simulink model "can_simple_block_bu11143"  (R2016b)
settings: Solver=FixedStepDiscrete  StartTime=0.0  StopTime=1000  FixedStep=0.2  RelTol=1e-3  EnableMultiTasking=on
undefined symbols (not defined in the file or in its folder): A, A10, A14, B, B11, B12, B13, B8, C, CS0, CS1, D, D11, D4, F3, F4, G, G3, G4, H3, H4, K17, K4, L3, N16, PA11, PA12, PD0, PE14, PE15, R10, R14, R17, SCK, SIN, SOUT, T14
libraries: rappid_564xl_ec_toolbox x59
(part 3 of 6)

== matlab function can_simple_block_bu11143/Function-Call Subsystem/Subsystem2/RawData to StoreData ==
  data: StrCell input; CellSOC_1_104 data_store_memory; VSOCDataCAN_8b output uint8
function VSOCDataCAN_8b = fcn(StrCell)

global CellSOC_1_104;
VSOCDataCAN_8b =  uint8(zeros(1,8));

      VSOCDataCAN_8b(1) =         CellSOC_1_104(StrCell*4-3)/256;
      VSOCDataCAN_8b(2) = mod(CellSOC_1_104(StrCell*4-3),256);
      VSOCDataCAN_8b(3) =         CellSOC_1_104(StrCell*4-2)/256;
      VSOCDataCAN_8b(4) = mod(CellSOC_1_104(StrCell*4-2),256);
      VSOCDataCAN_8b(5) =         CellSOC_1_104(StrCell*4-1)/256;
      VSOCDataCAN_8b(6) = mod(CellSOC_1_104(StrCell*4-1),256);
      VSOCDataCAN_8b(7) =         CellSOC_1_104(StrCell*4   )/256;
      VSOCDataCAN_8b(8) = mod(CellSOC_1_104(StrCell*4   ),256);

% VTDataCAN_8b(1) =         CellV_1_104(1)/256;
% VTDataCAN_8b(2) = mod(CellV_1_104(1),256);
% VTDataCAN_8b(3) =         CellV_1_104(2)/256;
% VTDataCAN_8b(4) = mod(CellV_1_104(2),256);
% VTDataCAN_8b(5) =         CellV_1_104(9)/256;
% VTDataCAN_8b(6) = mod(CellV_1_104(9),256);
% VTDataCAN_8b(7) =         CellV_1_104(10)/256;
% VTDataCAN_8b(8) = mod(CellV_1_104(10),256);

% VTDataCAN_8b(1) =         uint16(30000)/256;
% VTDataCAN_8b(2) = mod(uint16(30000),256);
% VTDataCAN_8b(3) =         uint16(35000)/256;
% VTDataCAN_8b(4) = mod(uint16(35000),256);
% VTDataCAN_8b(5) =         uint16(33000)/256;
% VTDataCAN_8b(6) = mod(uint16(33000),256);
% VTDataCAN_8b(7) =         uint16(20000)/256;
% VTDataCAN_8b(8) = mod(uint16(20000),256);


end








% CellV_1_104(1) = uint16(1);

% SPIDataStore = uint16(zeros(1,21));
% DataFault =  zeros(1,7);
%
% for i=1:7
%   SPIDataStore(i*3-2) = SPIData(i*8-7)+SPIData(i*8-6)*256;
%   SPIDataStore(i*3-1) = SPIData(i*8-5)+SPIData(i*8-4)*256;
%   SPIDataStore(i*3   ) = SPIData(i*8-3)+SPIData(i*8-2)*256;
%   if (PecChk(i*2-1) == SPIData(i*8-1)) && (PecChk(i*2) == SPIData(i*8))
%     DataFault(i) = 1;
%   else
%     DataFault(i) = 0;
%   end
% end



% onemask8 = uint16(hex2dec('00FF'));
% onemask8_8sft = uint16(hex2dec('FF00'));
% onemask88 = uint8(hex2dec('FF'));
% onemask16 = uint16(hex2dec('FFFF'));
%
% % data_test = zeros(1,2);
% remainder = uint16(16);
%
% for i=1:len
%     ii = uint16(i);
% %     data_test(1,i) = data(ii);
% %     address = 2;
%     address = bitand( ...
%         bitxor( ...
%         uint8(bitsra(remainder,7)),data(ii) ), ...
%         onemask88);
%     remainder = bitxor(bitshift(remainder,8,'uint16'),pec15Table(address+1));
% end
% pec15 = uint16(bitand(bitshift(remainder,1,'uint16'),onemask16));
% pec0 = uint8(bitand(pec15,onemask8));
% pec1 = uint8(bitsra(bitand(pec15,onemask8_8sft),8));

== stateflow chart can_simple_block_bu11143/Function-Call Subsystem/T_DUMP_CAN ==
  state A
    en: count = 0;
    du: count = count + 1;
  state A1
    en: count = 0;
  (default) -> A : {count =0;}
  A -> A1 : [count > count_in]{sig_trigger}
  A1 -> A
  data: count local double [0..10000]; count_in input
  events: sig_trigger output FUNCTION_CALL_EVENT

== stateflow chart can_simple_block_bu11143/Function-Call Subsystem/Subsystem4/Chart1 ==
  state A
    en: count  = count + 1;
    du: count = count + 1;
  state A1
    en: count = 1;
  (default) -> A : {count =0;}
  A1 -> A
  A -> A1 : [count >= count_in]
  data: count_in input; count output double [0..10000]

== matlab function can_simple_block_bu11143/Function-Call Subsystem/Subsystem4/RawData to StoreData ==
  data: StrCell input; CellGP_1_78 data_store_memory; VTDataCAN_8b output uint8
function VTDataCAN_8b = fcn(StrCell)

% global CellV_1_104;
global CellGP_1_78;
VTDataCAN_8b =  uint8(zeros(1,8));
% 
% StrCell_2 = fix((StrCell+1)/2);
% 
% if mod(StrCell,2)==1
% VTDataCAN_8b(1) =         CellGP_1_78(StrCell_2*6-5)/256;
% VTDataCAN_8b(2) = mod(CellGP_1_78(StrCell_2*6-5),256);
% VTDataCAN_8b(3) =         CellGP_1_78(StrCell_2*6-4)/256;
% VTDataCAN_8b(4) = mod(CellGP_1_78(StrCell_2*6-4),256);
% VTDataCAN_8b(5) =         CellGP_1_78(StrCell_2*6-3)/256;
% VTDataCAN_8b(6) = mod(CellGP_1_78(StrCell_2*6-3),256);
% VTDataCAN_8b(7) =         CellGP_1_78(StrCell_2*6-2 )/256;
% VTDataCAN_8b(8) = mod(CellGP_1_78(StrCell_2*6-2),256);
% else 
% VTDataCAN_8b(1) =         CellGP_1_78(StrCell_2*6-1 )/256;
% VTDataCAN_8b(2) = mod(CellGP_1_78(StrCell_2*6-1 ),256);
% VTDataCAN_8b(3) =         CellGP_1_78(StrCell_2*6-0 )/256;
% VTDataCAN_8b(4) = mod(CellGP_1_78(StrCell_2*6-0 ),256);
% end
onemask8 = uint16(hex2dec('00FF'));
onemask8_8sft = uint16(hex2dec('FF00'));
onemask8_56sft = uint64(hex2dec('FF'));
VTDataCAN_8b =  uint8(zeros(1,8));
VTDataCAN_64b =  uint64(zeros(1,1));
VTDataCAN_4data =  uint8(zeros(1,4));

Bid = StrCell;
VTDataCAN_64b = uint64( Bid ) + ...
                            uint64( bitshift(uint64(CellGP_1_78(StrCell*6-5)/64),8 ) ) + ...
                            uint64( bitshift(uint64(CellGP_1_78(StrCell*6-4)/64),8+10*1 ) )  + ...
                            uint64( bitshift(uint64(CellGP_1_78(StrCell*6-3)/64),8+10*2 ) )  + ...
                            uint64( bitshift(uint64(CellGP_1_78(StrCell*6-2)/64),8+10*3 ) ) + ...
                            uint64( bitshift(uint64(CellGP_1_78(StrCell*6-1)/64),8+10*4 ) ) + ...
                            uint64( bitshift(uint64(CellGP_1_78(StrCell*6-0)/1024),8+10*5 ) ) ;

VTDataCAN_8b(1) = uint8( bitand(VTDataCAN_64b,onemask8_56sft) );
VTDataCAN_8b(2) = uint8( bitand(bitsra(VTDataCAN_64b,8*1),onemask8_56sft) );
VTDataCAN_8b(3) = uint8( bitand(bitsra(VTDataCAN_64b,8*2),onemask8_56sft) );
VTDataCAN_8b(4) = uint8( bitand(bitsra(VTDataCAN_64b,8*3),onemask8_56sft) );
VTDataCAN_8b(5) = uint8( bitand(bitsra(VTDataCAN_64b,8*4),onemask8_56sft) );
VTDataCAN_8b(6) = uint8( bitand(bitsra(VTDataCAN_64b,8*5),onemask8_56sft) );
VTDataCAN_8b(7) = uint8( bitand(bitsra(VTDataCAN_64b,8*6),onemask8_56sft) );
VTDataCAN_8b(8) = uint8( bitand(bitsra(VTDataCAN_64b,8*7),onemask8_56sft) );


% VTDataCAN_8b(1) =         CellV_1_104(1)/256;
% VTDataCAN_8b(2) = mod(CellV_1_104(1),256);
% VTDataCAN_8b(3) =         CellV_1_104(2)/256;
% VTDataCAN_8b(4) = mod(CellV_1_104(2),256);
% VTDataCAN_8b(5) =         CellV_1_104(9)/256;
% VTDataCAN_8b(6) = mod(CellV_1_104(9),256);
% VTDataCAN_8b(7) =         CellV_1_104(10)/256;
% VTDataCAN_8b(8) = mod(CellV_1_104(10),256);

% VTDataCAN_8b(1) =         uint16(30000)/256;
% VTDataCAN_8b(2) = mod(uint16(30000),256);
% VTDataCAN_8b(3) =         uint16(35000)/256;
% VTDataCAN_8b(4) = mod(uint16(35000),256);
% VTDataCAN_8b(5) =         uint16(33000)/256;
% VTDataCAN_8b(6) = mod(uint16(33000),256);
% VTDataCAN_8b(7) =         uint16(20000)/256;
% VTDataCAN_8b(8) = mod(uint16(20000),256);


end








% CellV_1_104(1) = uint16(1);

% SPIDataStore = uint16(zeros(1,21));
% DataFault =  zeros(1,7);
%
% for i=1:7
%   SPIDataStore(i*3-2) = SPIData(i*8-7)+SPIData(i*8-6)*256;
%   SPIDataStore(i*3-1) = SPIData(i*8-5)+SPIData(i*8-4)*256;
%   SPIDataStore(i*3   ) = SPIData(i*8-3)+SPIData(i*8-2)*256;
%   if (PecChk(i*2-1) == SPIData(i*8-1)) && (PecChk(i*2) == SPIData(i*8))
%     DataFault(i) = 1;
%   else
%     DataFault(i) = 0;
%   end
% end



% onemask8 = uint16(hex2dec('00FF'));
% onemask8_8sft = uint16(hex2dec('FF00'));
% onemask88 = uint8(hex2dec('FF'));
% onemask16 = uint16(hex2dec('FFFF'));
%
% % data_test = zeros(1,2);
% remainder = uint16(16);
%
% for i=1:len
%     ii = uint16(i);
% %     data_test(1,i) = data(ii);
% %     address = 2;
%     address = bitand( ...
%         bitxor( ...
%         uint8(bitsra(remainder,7)),data(ii) ), ...
%         onemask88);
%     remainder = bitxor(bitshift(remainder,8,'uint16'),pec15Table(address+1));
% end
% pec15 = uint16(bitand(bitshift(remainder,1,'uint16'),onemask16));
% pec0 = uint8(bitand(pec15,onemask8));
% pec1 = uint8(bitsra(bitand(pec15,onemask8_8sft),8));

== matlab function can_simple_block_bu11143/Function-Call Subsystem/RawData to StoreData (SPICh1) ==
  data: STATE input; SPIData input; PecChk input; CellV_1_104 data_store_memory; DataFault output; CellGP_1_78 data_store_memory; V_REF_AUX data_store_memory
function DataFault   = fcnSpiCh1(STATE, SPIData, PecChk)

global CellV_1_104;
global CellGP_1_78;
global V_REF_AUX;
DataFault =  zeros(1,7);

% const int thermistor_ohm_table[231] = {//unit = 0.1Ohm
%                 36850000, 33710000, 30860000, 28270000, 25920000, 23780000, 21820000, 20050000, 18430000, 16950000, // -80 to -71 degC
%                 15600000, 14360000, 13230000, 12200000, 11260000, 10390000,  9599000,  8872000,  8205000,  7592000, // -70 to -61 degC
%                 7029000,  6511000,  6035000,  5597000,  5194000,  4822000,  4479000,  4163000,  3871000,  3602000, // -60 to -51 degC
%                 3353000,  3123000,  2910000,  2713000,  2530000,  2362000,  2205000,  2059000,  1925000,  1800000, // -50 to -41 degC
%                 2398000,  2260000,  2132000,  2011000,  1898000,  1792000,  1693000,  1600000,  1512000,  1430000, // -40 to -31 degC
%                 1352000,  1279000,  1211000,  1146000,  1086000,  1029000,   974900,   924300,   876600,   831600, // -30 to -21 degC
%                   789100,   749100,   711300,   675700,   642000,   610200,   580100,   551700,   524800,   499400, // -20 to -11 degC
%                   475400,   452700,   431100,   410700,   391400,   373100,   355700,   339300,   323700,   308900, // -10 to  -1 degC
%                   294900,   281500,   268900,   256900,   245500,   234600,   224300,   214500,   205200,   196300, //   0 to   9 degC
%                   187900,   179800,   172200,   164900,   157900,   151300,   145000,   139000,   133300,   127900, //  10 to  19 degC
%                   122600,   117700,   112900,   108400,   104100,   100000,    96050,    92270,    88670,    85230, //  20 to  29 degC
%                    81940,    78800,    75790,    72910,    70160,    67520,    65000,    62580,    60260,    58050, //  30 to  39 degC
%                    55920,    53890,    51930,    50060,    48270,    46550,    44890,    43310,    41790,    40330, //  40 to  49 degC
%                    38930,    37580,    36290,    35040,    33850,    32700,    31600,    30540,    29520,    28540, //  50 to  59 degC
%                    27600,    26690,    25820,    24970,    24170,    23390,    22640,    21910,    21220,    20550, //  60 to  69 degC
%                    19900,    19280,    18680,    18100,    17540,    17000,    16480,    15980,    15490,    15030, //  70 to  79 degC
%                    14580,    14140,    13720,    13320,    12930,    12550,    12180,    11830,    11400,    11160, //  80 to  89 degC
%                    10840,    10530,    10230,     9942,     9663,     9393,     9132,     8879,     8634,     8397, //  90 to  99 degC
%                     8168,     7946,     7731,     7523,     7321,     7126,     6936,     6753,     6575,     6403, // 100 to 109 degC
%                     6235,     6073,     5916,     5764,     5616,     5473,     5334,     5199,     5068,     4941, // 110 to 119 degC
%                     4818,     4698,     4582,     4469,     4359,     4253,     4149,     4049,     3951,     3856, // 120 to 129 degC
%                     3764,     3674,     3587,     3503,     3420,     3340,     3263,     3187,     3113,     3042, // 130 to 139 degC
%                     2972,     2904,     2838,     2774,     2712,     2651,     2592,     2534,     2478,     2423, // 140 to 149 degC
%                     2370                                                                                                                                                                                                                                                                                                                                                                  // 150        degC
% };

thermistor_ohm_table = 0.1*[
                36850000, 33710000, 30860000, 28270000, 25920000, 23780000, 21820000, 20050000, 18430000, 16950000, ...// -80 to -71 degC
                15600000, 14360000, 13230000, 12200000, 11260000, 10390000,  9599000,  8872000,  8205000,  7592000, ...// -70 to -61 degC
                7029000,  6511000,  6035000,  5597000,  5194000,  4822000,  4479000,  4163000,  3871000,  3602000, ...// -60 to -51 degC
                3353000,  3123000,  2910000,  2713000,  2530000,  2362000,  2205000,  2059000,  1925000,  1800000, ...// -50 to -41 degC
                2398000,  2260000,  2132000,  2011000,  1898000,  1792000,  1693000,  1600000,  1512000,  1430000, ...// -40 to -31 degC
                1352000,  1279000,  1211000,  1146000,  1086000,  1029000,   974900,   924300,   876600,   831600, ...// -30 to -21 degC
                  789100,   749100,   711300,   675700,   642000,   610200,   580100,   551700,   524800,   499400, ...// -20 to -11 degC
                  475400,   452700,   431100,   410700,   391400,   373100,   355700,   339300,   323700,   308900, ...// -10 to  -1 degC
                  294900,   281500,   268900,   256900,   245500,   234600,   224300,   214500,   205200,   196300, ...//   0 to   9 degC
                  187900,   179800,   172200,   164900,   157900,   151300,   145000,   139000,   133300,   127900, ...//  10 to  19 degC
                  122600,   117700,   112900,   108400,   104100,   100000,    96050,    92270,    88670,    85230,  ...//  20 to  29 degC
                   81940,    78800,    75790,    72910,    70160,    67520,    65000,    62580,    60260,    58050, ...//  30 to  39 degC
                   55920,    53890,    51930,    50060,    48270,    46550,    44890,    43310,    41790,    40330, ...//  40 to  49 degC
                   38930,    37580,    36290,    35040,    33850,    32700,    31600,    30540,    29520,    28540, ...//  50 to  59 degC
                   27600,    26690,    25820,    24970,    24170,    23390,    22640,    21910,    21220,    20550, ...//  60 to  69 degC
                   19900,    19280,    18680,    18100,    17540,    17000,    16480,    15980,    15490,    15030, ...//  70 to  79 degC
                   14580,    14140,    13720,    13320,    12930,    12550,    12180,    11830,    11400,    11160, ...//  80 to  89 degC
                   10840,    10530,    10230,     9942,     9663,     9393,     9132,     8879,     8634,     8397, ...//  90 to  99 degC
                    8168,     7946,     7731,     7523,     7321,     7126,     6936,     6753,     6575,     6403, ...// 100 to 109 degC
                    6235,     6073,     5916,     5764,     5616,     5473,     5334,     5199,     5068,     4941, ...// 110 to 119 degC
                    4818,     4698,     4582,     4469,     4359,     4253,     4149,     4049,     3951,     3856, ...// 120 to 129 degC
                    3764,     3674,     3587,     3503,     3420,     3340,     3263,     3187,     3113,     3042, ...// 130 to 139 degC
                    2972,     2904,     2838,     2774,     2712,     2651,     2592,     2534,     2478,     2423, ...// 140 to 149 degC
                     2370   ]; % // 150        degC



switch STATE
  case 0 % VC123
    for i=8:13
      CellV_1_104(i*8-7) = uint16(SPIData(i*8-7))+uint16(SPIData(i*8-6))*256;
      CellV_1_104(i*8-6) = uint16(SPIData(i*8-5))+uint16(SPIData(i*8-4))*256;
      CellV_1_104(i*8-5) = uint16(SPIData(i*8-3))+uint16(SPIData(i*8-2))*256;
      if (PecChk(i*2-1) == SPIData(i*8-1)) && (PecChk(i*2) == SPIData(i*8))
        DataFault(i) = 1;
      else
        DataFault(i) = 0;
      end
    end
  case 1 % VC456
    for i=8:13
      CellV_1_104(i*8-4) = uint16(SPIData(i*8-7))+uint16(SPIData(i*8-6))*256;
      CellV_1_104(i*8-3) = uint16(SPIData(i*8-5))+uint16(SPIData(i*8-4))*256;
      CellV_1_104(i*8-2) = uint16(SPIData(i*8-3))+uint16(SPIData(i*8-2))*256;
      if (PecChk(i*2-1) == SPIData(i*8-1)) && (PecChk(i*2) == SPIData(i*8))
        DataFault(i) = 1;
      else
        DataFault(i) = 0;
      end
    end    
  case 2 % VC78
    for i=8:13
      CellV_1_104(i*8-1) = uint16(SPIData(i*8-7))+uint16(SPIData(i*8-6))*256;
      CellV_1_104(i*8-0) = uint16(SPIData(i*8-5))+uint16(SPIData(i*8-4))*256;
%       CellV_1_104(i*8-2) = uint16(SPIData(i*8-3))+uint16(SPIData(i*8-2))*256;
      if (PecChk(i*2-1) == SPIData(i*8-1)) && (PecChk(i*2) == SPIData(i*8))
        DataFault(i) = 1;
      else
        DataFault(i) = 0;
      end
    end    
  case 3 % GP123
    for i=8:13
%       v_aux  = int16(uint16(SPIData(i*8-7))+uint16(SPIData(i*8-6))*256);
      v_aux  = (uint16(SPIData(i*8-7))+uint16(SPIData(i*8-6))*256);
      r_tm = (10000*v_aux)/(V_REF_AUX - v_aux);
       
       V_REF_AUX = uint16(30000);
      temperature = (find(thermistor_ohm_table<r_tm,1))-81;
      CellGP_1_78(i*6-5) = V_REF_AUX;
      
      v_aux  = (uint16(SPIData(i*8-5))+uint16(SPIData(i*8-4))*256);
      r_tm = (10000*v_aux)/(V_REF_AUX - v_aux);
      temperature = (find(thermistor_ohm_table<r_tm,1))-81;
       v_aux  = uint16(16000);       
      CellGP_1_78(i*6-4) = v_aux;
      
      v_aux  = (uint16(SPIData(i*8-3))+uint16(SPIData(i*8-2))*256);
      r_tm = (10000*v_aux) / (V_REF_AUX - v_aux);
      temperature = (find(thermistor_ohm_table<r_tm,1))-81;
      CellGP_1_78(i*6-3) = r_tm;      
      if (PecChk(i*2-1) == SPIData(i*8-1)) && (PecChk(i*2) == SPIData(i*8))
        DataFault(i) = 1;
      else
        DataFault(i) = 0;
      end
    end        
  case 4 % GP45
    for i=8:13
      v_aux  = (uint16(SPIData(i*8-7))+uint16(SPIData(i*8-6))*256);
      r_tm = (10000*v_aux)/(V_REF_AUX - v_aux);
      temperature = (find(thermistor_ohm_table<r_tm,1))-81;
      CellGP_1_78(i*6-2) = temperature;
      
      v_aux  = (uint16(SPIData(i*8-5))+uint16(SPIData(i*8-4))*256);
      r_tm = (10000*v_aux)/(V_REF_AUX - v_aux);
      temperature = (find(thermistor_ohm_table<r_tm,1))-81;
      CellGP_1_78(i*6-1) = temperature;      
      
      CellGP_1_78(i*6-0) = uint16(uint16(SPIData(i*8-3))+uint16(SPIData(i*8-2))*256);
      
      V_REF_AUX = (uint16(SPIData(i*8-3))+uint16(SPIData(i*8-2))*256);
      
      if (PecChk(i*2-1) == SPIData(i*8-1)) && (PecChk(i*2) == SPIData(i*8))
        DataFault(i) = 1;
      else
        DataFault(i) = 0;
      end
    end           
  otherwise % ERROR    
end


% CellV_1_104(1) = uint16(1);

% SPIDataStore = uint16(zeros(1,21));
% DataFault =  zeros(1,7);
%
% for i=1:7
%   SPIDataStore(i*3-2) = SPIData(i*8-7)+SPIData(i*8-6)*256;
%   SPIDataStore(i*3-1) = SPIData(i*8-5)+SPIData(i*8-4)*256;
%   SPIDataStore(i*3   ) = SPIData(i*8-3)+SPIData(i*8-2)*256;
%   if (PecChk(i*2-1) == SPIData(i*8-1)) && (PecChk(i*2) == SPIData(i*8))
%     DataFault(i) = 1;
%   else
%     DataFault(i) = 0;
%   end
% end



% onemask8 = uint16(hex2dec('00FF'));
% onemask8_8sft = uint16(hex2dec('FF00'));
% onemask88 = uint8(hex2dec('FF'));
% onemask16 = uint16(hex2dec('FFFF'));
%
% % data_test = zeros(1,2);
% remainder = uint16(16);
%
% for i=1:len
%     ii = uint16(i);
% %     data_test(1,i) = data(ii);
% %     address = 2;
%     address = bitand( ...
%         bitxor( ...
%         uint8(bitsra(remainder,7)),data(ii) ), ...
%         onemask88);
%     remainder = bitxor(bitshift(remainder,8,'uint16'),pec15Table(address+1));
% end
% pec15 = uint16(bitand(bitshift(remainder,1,'uint16'),onemask16));
% pec0 = uint8(bitand(pec15,onemask8));
% pec1 = uint8(bitsra(bitand(pec15,onemask8_8sft),8));

== matlab function can_simple_block_bu11143/DataDumpFast1/RawData to StoreData2 ==
  data: StrCell input; CellV_1_104 data_store_memory; VTDataCAN_8b output uint8
function VTDataCAN_8b = fcn(StrCell)
global CellV_1_104;
onemask8 = uint16(hex2dec('00FF'));
onemask8_8sft = uint16(hex2dec('FF00'));
onemask8_56sft = uint64(hex2dec('FF'));
% yl = uint8(bitand(u,onemask8));
% yh = uint8(bitsra(bitand(u,onemask8_8sft),8));
% bitshift(remainder,8)  shift left
% bitsra(remainder,8)  shift right



VTDataCAN_8b =  uint8(zeros(1,8));
VTDataCAN_64b =  uint64(zeros(1,1));
VTDataCAN_4data =  uint8(zeros(1,4));

% VTDataCAN_4data(1) = fix(CellV_1_104(StrCell*4-3)/4);
% VTDataCAN_4data(2) = fix(CellV_1_104(StrCell*4-2)/4);
% VTDataCAN_4data(3) = fix(CellV_1_104(StrCell*4-1)/4);
% VTDataCAN_4data(4) = fix(CellV_1_104(StrCell*4-0)/4);

Bid = StrCell;
VTDataCAN_64b = uint64( Bid ) + ...
                            uint64( bitshift(uint64(CellV_1_104(StrCell*4-3)/4),8 ) ) + ...
                            uint64( bitshift(uint64(CellV_1_104(StrCell*4-2)/4),8+14 ))  + ...
                            uint64( bitshift(uint64(CellV_1_104(StrCell*4-1)/4),8+14+14)  )  + ...
                            uint64( bitshift(uint64(CellV_1_104(StrCell*4-0)/4),8+14+14+14) ) ;

VTDataCAN_8b(1) = uint8( bitand(VTDataCAN_64b,onemask8_56sft) );
VTDataCAN_8b(2) = uint8( bitand(bitsra(VTDataCAN_64b,8*1),onemask8_56sft) );
VTDataCAN_8b(3) = uint8( bitand(bitsra(VTDataCAN_64b,8*2),onemask8_56sft) );
VTDataCAN_8b(4) = uint8( bitand(bitsra(VTDataCAN_64b,8*3),onemask8_56sft) );
VTDataCAN_8b(5) = uint8( bitand(bitsra(VTDataCAN_64b,8*4),onemask8_56sft) );
VTDataCAN_8b(6) = uint8( bitand(bitsra(VTDataCAN_64b,8*5),onemask8_56sft) );
VTDataCAN_8b(7) = uint8( bitand(bitsra(VTDataCAN_64b,8*6),onemask8_56sft) );
VTDataCAN_8b(8) = uint8( bitand(bitsra(VTDataCAN_64b,8*7),onemask8_56sft) );

% VTDataCAN_8b(1) = Bid;
% VTDataCAN_8b(2) = VTDataCAN_4data(1)/(2^8);
% VTDataCAN_8b(3) = 4*fix(mod(CellV_1_104(StrCell*4-3),2^8)/4);
% VTDataCAN_8b(3) = VTDataCAN_8b(3) + CellV_1_104(StrCell*4-2)/(2^14);
% VTDataCAN_8b(4) = mod(CellV_1_104(StrCell*4-2),2^14) / (2^8);
% VTDataCAN_8b(5) =  * fix(mod(CellV_1_104(StrCell*4-2),2^6));

4*fix(CellV_1_104(StrCell*4-3)/4);


% VTDataCAN_8b(1) =         CellV_1_104(StrCell*4-3)/256;
% VTDataCAN_8b(2) = mod(CellV_1_104(StrCell*4-3),256);
% VTDataCAN_8b(3) =         CellV_1_104(StrCell*4-2)/256;
% VTDataCAN_8b(4) = mod(CellV_1_104(StrCell*4-2),256);
% VTDataCAN_8b(5) =         CellV_1_104(StrCell*4-1)/256;
% VTDataCAN_8b(6) = mod(CellV_1_104(StrCell*4-1),256);
% VTDataCAN_8b(7) =         CellV_1_104(StrCell*4   )/256;
% VTDataCAN_8b(8) = mod(CellV_1_104(StrCell*4   ),256);

% VTDataCAN_8b(1) =         CellV_1_104(1)/256;
% VTDataCAN_8b(2) = mod(CellV_1_104(1),256);
% VTDataCAN_8b(3) =         CellV_1_104(2)/256;
% VTDataCAN_8b(4) = mod(CellV_1_104(2),256);
% VTDataCAN_8b(5) =         CellV_1_104(9)/256;
% VTDataCAN_8b(6) = mod(CellV_1_104(9),256);
% VTDataCAN_8b(7) =         CellV_1_104(10)/256;
% VTDataCAN_8b(8) = mod(CellV_1_104(10),256);

% VTDataCAN_8b(1) =         uint16(30000)/256;
% VTDataCAN_8b(2) = mod(uint16(30000),256);
% VTDataCAN_8b(3) =         uint16(35000)/256;
% VTDataCAN_8b(4) = mod(uint16(35000),256);
% VTDataCAN_8b(5) =         uint16(33000)/256;
% VTDataCAN_8b(6) = mod(uint16(33000),256);
% VTDataCAN_8b(7) =         uint16(20000)/256;
% VTDataCAN_8b(8) = mod(uint16(20000),256);


end








% CellV_1_104(1) = uint16(1);

% SPIDataStore = uint16(zeros(1,21));
% DataFault =  zeros(1,7);
%
% for i=1:7
%   SPIDataStore(i*3-2) = SPIData(i*8-7)+SPIData(i*8-6)*256;
%   SPIDataStore(i*3-1) = SPIData(i*8-5)+SPIData(i*8-4)*256;
%   SPIDataStore(i*3   ) = SPIData(i*8-3)+SPIData(i*8-2)*256;
%   if (PecChk(i*2-1) == SPIData(i*8-1)) && (PecChk(i*2) == SPIData(i*8))
%     DataFault(i) = 1;
%   else
%     DataFault(i) = 0;
%   end
% end



% onemask8 = uint16(hex2dec('00FF'));
% onemask8_8sft = uint16(hex2dec('FF00'));
% onemask88 = uint8(hex2dec('FF'));
% onemask16 = uint16(hex2dec('FFFF'));
%
% % data_test = zeros(1,2);
% remainder = uint16(16);
%
% for i=1:len
%     ii = uint16(i);
% %     data_test(1,i) = data(ii);
% %     address = 2;
%     address = bitand( ...
%         bitxor( ...
%         uint8(bitsra(remainder,7)),data(ii) ), ...
%         onemask88);
%     remainder = bitxor(bitshift(remainder,8,'uint16'),pec15Table(address+1));
% end
% pec15 = uint16(bitand(bitshift(remainder,1,'uint16'),onemask16));
% pec0 = uint8(bitand(pec15,onemask8));
% pec1 = uint8(bitsra(bitand(pec15,onemask8_8sft),8));

== stateflow chart can_simple_block_bu11143/DataDumpFast1/Chart2 ==
  state A
    en: count  = count + 1;
    du: count = count + 1;
  state A1
    en: count = 1;
  (default) -> A : {count =0;}
  A1 -> A
  A -> A1 : [count >= count_in]
  data: count_in input; count output double [0..10000]

== matlab function can_simple_block_bu11143/DataDumpFast1/RawData to StoreData ==
  data: StrCell input; CellV_1_104 data_store_memory; VTDataCAN_8b output uint8
function VTDataCAN_8b = fcn(StrCell)
global CellV_1_104;
onemask8 = uint16(hex2dec('00FF'));
onemask8_8sft = uint16(hex2dec('FF00'));
onemask8_56sft = uint64(hex2dec('FF'));
% yl = uint8(bitand(u,onemask8));
% yh = uint8(bitsra(bitand(u,onemask8_8sft),8));
% bitshift(remainder,8)  shift left
% bitsra(remainder,8)  shift right



VTDataCAN_8b =  uint8(zeros(1,8));
VTDataCAN_64b =  uint64(zeros(1,1));
VTDataCAN_4data =  uint8(zeros(1,4));

% VTDataCAN_4data(1) = fix(CellV_1_104(StrCell*4-3)/4);
% VTDataCAN_4data(2) = fix(CellV_1_104(StrCell*4-2)/4);
% VTDataCAN_4data(3) = fix(CellV_1_104(StrCell*4-1)/4);
% VTDataCAN_4data(4) = fix(CellV_1_104(StrCell*4-0)/4);

Bid = StrCell;
VTDataCAN_64b = uint64( Bid ) + ...
                            uint64( bitshift(uint64(CellV_1_104(StrCell*4-3)/4),8 ) ) + ...
                            uint64( bitshift(uint64(CellV_1_104(StrCell*4-2)/4),8+14 ))  + ...
                            uint64( bitshift(uint64(CellV_1_104(StrCell*4-1)/4),8+14+14)  )  + ...
                            uint64( bitshift(uint64(CellV_1_104(StrCell*4-0)/4),8+14+14+14) ) ;

VTDataCAN_8b(1) = uint8( bitand(VTDataCAN_64b,onemask8_56sft) );
VTDataCAN_8b(2) = uint8( bitand(bitsra(VTDataCAN_64b,8*1),onemask8_56sft) );
VTDataCAN_8b(3) = uint8( bitand(bitsra(VTDataCAN_64b,8*2),onemask8_56sft) );
VTDataCAN_8b(4) = uint8( bitand(bitsra(VTDataCAN_64b,8*3),onemask8_56sft) );
VTDataCAN_8b(5) = uint8( bitand(bitsra(VTDataCAN_64b,8*4),onemask8_56sft) );
VTDataCAN_8b(6) = uint8( bitand(bitsra(VTDataCAN_64b,8*5),onemask8_56sft) );
VTDataCAN_8b(7) = uint8( bitand(bitsra(VTDataCAN_64b,8*6),onemask8_56sft) );
VTDataCAN_8b(8) = uint8( bitand(bitsra(VTDataCAN_64b,8*7),onemask8_56sft) );

% VTDataCAN_8b(1) = Bid;
% VTDataCAN_8b(2) = VTDataCAN_4data(1)/(2^8);
% VTDataCAN_8b(3) = 4*fix(mod(CellV_1_104(StrCell*4-3),2^8)/4);
% VTDataCAN_8b(3) = VTDataCAN_8b(3) + CellV_1_104(StrCell*4-2)/(2^14);
% VTDataCAN_8b(4) = mod(CellV_1_104(StrCell*4-2),2^14) / (2^8);
% VTDataCAN_8b(5) =  * fix(mod(CellV_1_104(StrCell*4-2),2^6));

4*fix(CellV_1_104(StrCell*4-3)/4);


% VTDataCAN_8b(1) =         CellV_1_104(StrCell*4-3)/256;
% VTDataCAN_8b(2) = mod(CellV_1_104(StrCell*4-3),256);
% VTDataCAN_8b(3) =         CellV_1_104(StrCell*4-2)/256;
% VTDataCAN_8b(4) = mod(CellV_1_104(StrCell*4-2),256);
% VTDataCAN_8b(5) =         CellV_1_104(StrCell*4-1)/256;
% VTDataCAN_8b(6) = mod(CellV_1_104(StrCell*4-1),256);
% VTDataCAN_8b(7) =         CellV_1_104(StrCell*4   )/256;
% VTDataCAN_8b(8) = mod(CellV_1_104(StrCell*4   ),256);

% VTDataCAN_8b(1) =         CellV_1_104(1)/256;
% VTDataCAN_8b(2) = mod(CellV_1_104(1),256);
% VTDataCAN_8b(3) =         CellV_1_104(2)/256;
% VTDataCAN_8b(4) = mod(CellV_1_104(2),256);
% VTDataCAN_8b(5) =         CellV_1_104(9)/256;
% VTDataCAN_8b(6) = mod(CellV_1_104(9),256);
% VTDataCAN_8b(7) =         CellV_1_104(10)/256;
% VTDataCAN_8b(8) = mod(CellV_1_104(10),256);

% VTDataCAN_8b(1) =         uint16(30000)/256;
% VTDataCAN_8b(2) = mod(uint16(30000),256);
% VTDataCAN_8b(3) =         uint16(35000)/256;
% VTDataCAN_8b(4) = mod(uint16(35000),256);
% VTDataCAN_8b(5) =         uint16(33000)/256;
% VTDataCAN_8b(6) = mod(uint16(33000),256);
% VTDataCAN_8b(7) =         uint16(20000)/256;
% VTDataCAN_8b(8) = mod(uint16(20000),256);


end








% CellV_1_104(1) = uint16(1);

% SPIDataStore = uint16(zeros(1,21));
% DataFault =  zeros(1,7);
%
% for i=1:7
%   SPIDataStore(i*3-2) = SPIData(i*8-7)+SPIData(i*8-6)*256;
%   SPIDataStore(i*3-1) = SPIData(i*8-5)+SPIData(i*8-4)*256;
%   SPIDataStore(i*3   ) = SPIData(i*8-3)+SPIData(i*8-2)*256;
%   if (PecChk(i*2-1) == SPIData(i*8-1)) && (PecChk(i*2) == SPIData(i*8))
%     DataFault(i) = 1;
%   else
%     DataFault(i) = 0;
%   end
% end



% onemask8 = uint16(hex2dec('00FF'));
% onemask8_8sft = uint16(hex2dec('FF00'));
% onemask88 = uint8(hex2dec('FF'));
% onemask16 = uint16(hex2dec('FFFF'));
%
% % data_test = zeros(1,2);
% remainder = uint16(16);
%
% for i=1:len
%     ii = uint16(i);
% %     data_test(1,i) = data(ii);
% %     address = 2;
%     address = bitand( ...
%         bitxor( ...
%         uint8(bitsra(remainder,7)),data(ii) ), ...
%         onemask88);
%     remainder = bitxor(bitshift(remainder,8,'uint16'),pec15Table(address+1));
% end
% pec15 = uint16(bitand(bitshift(remainder,1,'uint16'),onemask16));
% pec0 = uint8(bitand(pec15,onemask8));
% pec1 = uint8(bitsra(bitand(pec15,onemask8_8sft),8));

== matlab function can_simple_block_bu11143/DataDumpFast1/RawData to StoreData1 ==
  data: StrCell input; CellGP_1_78 data_store_memory; VTDataCAN_8b output uint8
function VTDataCAN_8b = fcn(StrCell)

% global CellV_1_104;
global CellGP_1_78;
VTDataCAN_8b =  uint8(zeros(1,8));
% 
% StrCell_2 = fix((StrCell+1)/2);
% 
% if mod(StrCell,2)==1
% VTDataCAN_8b(1) =         CellGP_1_78(StrCell_2*6-5)/256;
% VTDataCAN_8b(2) = mod(CellGP_1_78(StrCell_2*6-5),256);
% VTDataCAN_8b(3) =         CellGP_1_78(StrCell_2*6-4)/256;
% VTDataCAN_8b(4) = mod(CellGP_1_78(StrCell_2*6-4),256);
% VTDataCAN_8b(5) =         CellGP_1_78(StrCell_2*6-3)/256;
% VTDataCAN_8b(6) = mod(CellGP_1_78(StrCell_2*6-3),256);
% VTDataCAN_8b(7) =         CellGP_1_78(StrCell_2*6-2 )/256;
% VTDataCAN_8b(8) = mod(CellGP_1_78(StrCell_2*6-2),256);
% else 
% VTDataCAN_8b(1) =         CellGP_1_78(StrCell_2*6-1 )/256;
% VTDataCAN_8b(2) = mod(CellGP_1_78(StrCell_2*6-1 ),256);
% VTDataCAN_8b(3) =         CellGP_1_78(StrCell_2*6-0 )/256;
% VTDataCAN_8b(4) = mod(CellGP_1_78(StrCell_2*6-0 ),256);
% end
onemask8 = uint16(hex2dec('00FF'));
onemask8_8sft = uint16(hex2dec('FF00'));
onemask8_56sft = uint64(hex2dec('FF'));
VTDataCAN_8b =  uint8(zeros(1,8));
VTDataCAN_64b =  uint64(zeros(1,1));
VTDataCAN_4data =  uint8(zeros(1,4));

Bid = StrCell;
VTDataCAN_64b = uint64( Bid ) + ...
                            uint64( bitshift(uint64(CellGP_1_78(StrCell*6-5)/64),8 ) ) + ...
                            uint64( bitshift(uint64(CellGP_1_78(StrCell*6-4)/64),8+10*1 ) )  + ...
                            uint64( bitshift(uint64(CellGP_1_78(StrCell*6-3)/64),8+10*2 ) )  + ...
                            uint64( bitshift(uint64(CellGP_1_78(StrCell*6-2)/64),8+10*3 ) ) + ...
                            uint64( bitshift(uint64(CellGP_1_78(StrCell*6-1)/64),8+10*4 ) ) + ...
                            uint64( bitshift(uint64(CellGP_1_78(StrCell*6-0)/1024),8+10*5 ) ) ;

VTDataCAN_8b(1) = uint8( bitand(VTDataCAN_64b,onemask8_56sft) );
VTDataCAN_8b(2) = uint8( bitand(bitsra(VTDataCAN_64b,8*1),onemask8_56sft) );
VTDataCAN_8b(3) = uint8( bitand(bitsra(VTDataCAN_64b,8*2),onemask8_56sft) );
VTDataCAN_8b(4) = uint8( bitand(bitsra(VTDataCAN_64b,8*3),onemask8_56sft) );
VTDataCAN_8b(5) = uint8( bitand(bitsra(VTDataCAN_64b,8*4),onemask8_56sft) );
VTDataCAN_8b(6) = uint8( bitand(bitsra(VTDataCAN_64b,8*5),onemask8_56sft) );
VTDataCAN_8b(7) = uint8( bitand(bitsra(VTDataCAN_64b,8*6),onemask8_56sft) );
VTDataCAN_8b(8) = uint8( bitand(bitsra(VTDataCAN_64b,8*7),onemask8_56sft) );


% VTDataCAN_8b(1) =         CellV_1_104(1)/256;
% VTDataCAN_8b(2) = mod(CellV_1_104(1),256);
% VTDataCAN_8b(3) =         CellV_1_104(2)/256;
% VTDataCAN_8b(4) = mod(CellV_1_104(2),256);
% VTDataCAN_8b(5) =         CellV_1_104(9)/256;
% VTDataCAN_8b(6) = mod(CellV_1_104(9),256);
% VTDataCAN_8b(7) =         CellV_1_104(10)/256;
% VTDataCAN_8b(8) = mod(CellV_1_104(10),256);

% VTDataCAN_8b(1) =         uint16(30000)/256;
% VTDataCAN_8b(2) = mod(uint16(30000),256);
% VTDataCAN_8b(3) =         uint16(35000)/256;
% VTDataCAN_8b(4) = mod(uint16(35000),256);
% VTDataCAN_8b(5) =         uint16(33000)/256;
% VTDataCAN_8b(6) = mod(uint16(33000),256);
% VTDataCAN_8b(7) =         uint16(20000)/256;
% VTDataCAN_8b(8) = mod(uint16(20000),256);


end








% CellV_1_104(1) = uint16(1);

% SPIDataStore = uint16(zeros(1,21));
% DataFault =  zeros(1,7);
%
% for i=1:7
%   SPIDataStore(i*3-2) = SPIData(i*8-7)+SPIData(i*8-6)*256;
%   SPIDataStore(i*3-1) = SPIData(i*8-5)+SPIData(i*8-4)*256;
%   SPIDataStore(i*3   ) = SPIData(i*8-3)+SPIData(i*8-2)*256;
%   if (PecChk(i*2-1) == SPIData(i*8-1)) && (PecChk(i*2) == SPIData(i*8))
%     DataFault(i) = 1;
%   else
%     DataFault(i) = 0;
%   end
% end



% onemask8 = uint16(hex2dec('00FF'));
% onemask8_8sft = uint16(hex2dec('FF00'));
% onemask88 = uint8(hex2dec('FF'));
% onemask16 = uint16(hex2dec('FFFF'));
%
% % data_test = zeros(1,2);
% remainder = uint16(16);
%
% for i=1:len
%     ii = uint16(i);
% %     data_test(1,i) = data(ii);
% %     address = 2;
%     address = bitand( ...
%         bitxor( ...
%         uint8(bitsra(remainder,7)),data(ii) ), ...
%         onemask88);
%     remainder = bitxor(bitshift(remainder,8,'uint16'),pec15Table(address+1));
% end
% pec15 = uint16(bitand(bitshift(remainder,1,'uint16'),onemask16));
% pec0 = uint8(bitand(pec15,onemask8));
% pec1 = uint8(bitsra(bitand(pec15,onemask8_8sft),8));

== matlab function can_simple_block_bu11143/DataDumpFast1/RawData to StoreData3 ==
  data: StrCell input; CellV_1_104 data_store_memory; VTDataCAN_8b output uint8
function VTDataCAN_8b = fcn(StrCell)
global CellV_1_104;
onemask8 = uint16(hex2dec('00FF'));
onemask8_8sft = uint16(hex2dec('FF00'));
onemask8_56sft = uint64(hex2dec('FF'));
% yl = uint8(bitand(u,onemask8));
% yh = uint8(bitsra(bitand(u,onemask8_8sft),8));
% bitshift(remainder,8)  shift left
% bitsra(remainder,8)  shift right



VTDataCAN_8b =  uint8(zeros(1,8));
VTDataCAN_64b =  uint64(zeros(1,1));
VTDataCAN_4data =  uint8(zeros(1,4));

% VTDataCAN_4data(1) = fix(CellV_1_104(StrCell*4-3)/4);
% VTDataCAN_4data(2) = fix(CellV_1_104(StrCell*4-2)/4);
% VTDataCAN_4data(3) = fix(CellV_1_104(StrCell*4-1)/4);
% VTDataCAN_4data(4) = fix(CellV_1_104(StrCell*4-0)/4);

Bid = StrCell;
VTDataCAN_64b = uint64( Bid ) + ...
                            uint64( bitshift(uint64(CellV_1_104(StrCell*4-3)/4),8 ) ) + ...
                            uint64( bitshift(uint64(CellV_1_104(StrCell*4-2)/4),8+14 ))  + ...
                            uint64( bitshift(uint64(CellV_1_104(StrCell*4-1)/4),8+14+14)  )  + ...
                            uint64( bitshift(uint64(CellV_1_104(StrCell*4-0)/4),8+14+14+14) ) ;

VTDataCAN_8b(1) = uint8( bitand(VTDataCAN_64b,onemask8_56sft) );
VTDataCAN_8b(2) = uint8( bitand(bitsra(VTDataCAN_64b,8*1),onemask8_56sft) );
VTDataCAN_8b(3) = uint8( bitand(bitsra(VTDataCAN_64b,8*2),onemask8_56sft) );
VTDataCAN_8b(4) = uint8( bitand(bitsra(VTDataCAN_64b,8*3),onemask8_56sft) );
VTDataCAN_8b(5) = uint8( bitand(bitsra(VTDataCAN_64b,8*4),onemask8_56sft) );
VTDataCAN_8b(6) = uint8( bitand(bitsra(VTDataCAN_64b,8*5),onemask8_56sft) );
VTDataCAN_8b(7) = uint8( bitand(bitsra(VTDataCAN_64b,8*6),onemask8_56sft) );
VTDataCAN_8b(8) = uint8( bitand(bitsra(VTDataCAN_64b,8*7),onemask8_56sft) );

% VTDataCAN_8b(1) = Bid;
% VTDataCAN_8b(2) = VTDataCAN_4data(1)/(2^8);
% VTDataCAN_8b(3) = 4*fix(mod(CellV_1_104(StrCell*4-3),2^8)/4);
% VTDataCAN_8b(3) = VTDataCAN_8b(3) + CellV_1_104(StrCell*4-2)/(2^14);
% VTDataCAN_8b(4) = mod(CellV_1_104(StrCell*4-2),2^14) / (2^8);
% VTDataCAN_8b(5) =  * fix(mod(CellV_1_104(StrCell*4-2),2^6));

4*fix(CellV_1_104(StrCell*4-3)/4);


% VTDataCAN_8b(1) =         CellV_1_104(StrCell*4-3)/256;
% VTDataCAN_8b(2) = mod(CellV_1_104(StrCell*4-3),256);
% VTDataCAN_8b(3) =         CellV_1_104(StrCell*4-2)/256;
% VTDataCAN_8b(4) = mod(CellV_1_104(StrCell*4-2),256);
% VTDataCAN_8b(5) =         CellV_1_104(StrCell*4-1)/256;
% VTDataCAN_8b(6) = mod(CellV_1_104(StrCell*4-1),256);
% VTDataCAN_8b(7) =         CellV_1_104(StrCell*4   )/256;
% VTDataCAN_8b(8) = mod(CellV_1_104(StrCell*4   ),256);

% VTDataCAN_8b(1) =         CellV_1_104(1)/256;
% VTDataCAN_8b(2) = mod(CellV_1_104(1),256);
% VTDataCAN_8b(3) =         CellV_1_104(2)/256;
% VTDataCAN_8b(4) = mod(CellV_1_104(2),256);
% VTDataCAN_8b(5) =         CellV_1_104(9)/256;
% VTDataCAN_8b(6) = mod(CellV_1_104(9),256);
% VTDataCAN_8b(7) =         CellV_1_104(10)/256;
% VTDataCAN_8b(8) = mod(CellV_1_104(10),256);

% VTDataCAN_8b(1) =         uint16(30000)/256;
% VTDataCAN_8b(2) = mod(uint16(30000),256);
% VTDataCAN_8b(3) =         uint16(35000)/256;
% VTDataCAN_8b(4) = mod(uint16(35000),256);
% VTDataCAN_8b(5) =         uint16(33000)/256;
% VTDataCAN_8b(6) = mod(uint16(33000),256);
% VTDataCAN_8b(7) =         uint16(20000)/256;
% VTDataCAN_8b(8) = mod(uint16(20000),256);


end








% CellV_1_104(1) = uint16(1);

% SPIDataStore = uint16(zeros(1,21));
% DataFault =  zeros(1,7);
%
% for i=1:7
%   SPIDataStore(i*3-2) = SPIData(i*8-7)+SPIData(i*8-6)*256;
%   SPIDataStore(i*3-1) = SPIData(i*8-5)+SPIData(i*8-4)*256;
%   SPIDataStore(i*3   ) = SPIData(i*8-3)+SPIData(i*8-2)*256;
%   if (PecChk(i*2-1) == SPIData(i*8-1)) && (PecChk(i*2) == SPIData(i*8))
%     DataFault(i) = 1;
%   else
%     DataFault(i) = 0;
%   end
% end



% onemask8 = uint16(hex2dec('00FF'));
% onemask8_8sft = uint16(hex2dec('FF00'));
% onemask88 = uint8(hex2dec('FF'));
% onemask16 = uint16(hex2dec('FFFF'));
%
% % data_test = zeros(1,2);
% remainder = uint16(16);
%
% for i=1:len
%     ii = uint16(i);
% %     data_test(1,i) = data(ii);
% %     address = 2;
%     address = bitand( ...
%         bitxor( ...
%         uint8(bitsra(remainder,7)),data(ii) ), ...
%         onemask88);
%     remainder = bitxor(bitshift(remainder,8,'uint16'),pec15Table(address+1));
% end
% pec15 = uint16(bitand(bitshift(remainder,1,'uint16'),onemask16));
% pec0 = uint8(bitand(pec15,onemask8));
% pec1 = uint8(bitsra(bitand(pec15,onemask8_8sft),8));

== matlab function can_simple_block_bu11143/DataDumpFast1/RawData to StoreData4 ==
  data: StrCell input; CellV_1_104 data_store_memory; VTDataCAN_8b output uint8
function VTDataCAN_8b = fcn(StrCell)
global CellV_1_104;
onemask8 = uint16(hex2dec('00FF'));
onemask8_8sft = uint16(hex2dec('FF00'));
onemask8_56sft = uint64(hex2dec('FF'));
% yl = uint8(bitand(u,onemask8));
% yh = uint8(bitsra(bitand(u,onemask8_8sft),8));
% bitshift(remainder,8)  shift left
% bitsra(remainder,8)  shift right



VTDataCAN_8b =  uint8(zeros(1,8));
VTDataCAN_64b =  uint64(zeros(1,1));
VTDataCAN_4data =  uint8(zeros(1,4));

% VTDataCAN_4data(1) = fix(CellV_1_104(StrCell*4-3)/4);
% VTDataCAN_4data(2) = fix(CellV_1_104(StrCell*4-2)/4);
% VTDataCAN_4data(3) = fix(CellV_1_104(StrCell*4-1)/4);
% VTDataCAN_4data(4) = fix(CellV_1_104(StrCell*4-0)/4);

Bid = StrCell;
VTDataCAN_64b = uint64( Bid ) + ...
                            uint64( bitshift(uint64(CellV_1_104(StrCell*4-3)/4),8 ) ) + ...
                            uint64( bitshift(uint64(CellV_1_104(StrCell*4-2)/4),8+14 ))  + ...
                            uint64( bitshift(uint64(CellV_1_104(StrCell*4-1)/4),8+14+14)  )  + ...
                            uint64( bitshift(uint64(CellV_1_104(StrCell*4-0)/4),8+14+14+14) ) ;

VTDataCAN_8b(1) = uint8( bitand(VTDataCAN_64b,onemask8_56sft) );
VTDataCAN_8b(2) = uint8( bitand(bitsra(VTDataCAN_64b,8*1),onemask8_56sft) );
VTDataCAN_8b(3) = uint8( bitand(bitsra(VTDataCAN_64b,8*2),onemask8_56sft) );
VTDataCAN_8b(4) = uint8( bitand(bitsra(VTDataCAN_64b,8*3),onemask8_56sft) );
VTDataCAN_8b(5) = uint8( bitand(bitsra(VTDataCAN_64b,8*4),onemask8_56sft) );
VTDataCAN_8b(6) = uint8( bitand(bitsra(VTDataCAN_64b,8*5),onemask8_56sft) );
VTDataCAN_8b(7) = uint8( bitand(bitsra(VTDataCAN_64b,8*6),onemask8_56sft) );
VTDataCAN_8b(8) = uint8( bitand(bitsra(VTDataCAN_64b,8*7),onemask8_56sft) );

% VTDataCAN_8b(1) = Bid;
% VTDataCAN_8b(2) = VTDataCAN_4data(1)/(2^8);
% VTDataCAN_8b(3) = 4*fix(mod(CellV_1_104(StrCell*4-3),2^8)/4);
% VTDataCAN_8b(3) = VTDataCAN_8b(3) + CellV_1_104(StrCell*4-2)/(2^14);
% VTDataCAN_8b(4) = mod(CellV_1_104(StrCell*4-2),2^14) / (2^8);
% VTDataCAN_8b(5) =  * fix(mod(CellV_1_104(StrCell*4-2),2^6));

4*fix(CellV_1_104(StrCell*4-3)/4);


% VTDataCAN_8b(1) =         CellV_1_104(StrCell*4-3)/256;
% VTDataCAN_8b(2) = mod(CellV_1_104(StrCell*4-3),256);
% VTDataCAN_8b(3) =         CellV_1_104(StrCell*4-2)/256;
% VTDataCAN_8b(4) = mod(CellV_1_104(StrCell*4-2),256);
% VTDataCAN_8b(5) =         CellV_1_104(StrCell*4-1)/256;
% VTDataCAN_8b(6) = mod(CellV_1_104(StrCell*4-1),256);
% VTDataCAN_8b(7) =         CellV_1_104(StrCell*4   )/256;
% VTDataCAN_8b(8) = mod(CellV_1_104(StrCell*4   ),256);

% VTDataCAN_8b(1) =         CellV_1_104(1)/256;
% VTDataCAN_8b(2) = mod(CellV_1_104(1),256);
% VTDataCAN_8b(3) =         CellV_1_104(2)/256;
% VTDataCAN_8b(4) = mod(CellV_1_104(2),256);
% VTDataCAN_8b(5) =         CellV_1_104(9)/256;
% VTDataCAN_8b(6) = mod(CellV_1_104(9),256);
% VTDataCAN_8b(7) =         CellV_1_104(10)/256;
% VTDataCAN_8b(8) = mod(CellV_1_104(10),256);

% VTDataCAN_8b(1) =         uint16(30000)/256;
% VTDataCAN_8b(2) = mod(uint16(30000),256);
% VTDataCAN_8b(3) =         uint16(35000)/256;
% VTDataCAN_8b(4) = mod(uint16(35000),256);
% VTDataCAN_8b(5) =         uint16(33000)/256;
% VTDataCAN_8b(6) = mod(uint16(33000),256);
% VTDataCAN_8b(7) =         uint16(20000)/256;
% VTDataCAN_8b(8) = mod(uint16(20000),256);


end








% CellV_1_104(1) = uint16(1);

% SPIDataStore = uint16(zeros(1,21));
% DataFault =  zeros(1,7);
%
% for i=1:7
%   SPIDataStore(i*3-2) = SPIData(i*8-7)+SPIData(i*8-6)*256;
%   SPIDataStore(i*3-1) = SPIData(i*8-5)+SPIData(i*8-4)*256;
%   SPIDataStore(i*3   ) = SPIData(i*8-3)+SPIData(i*8-2)*256;
%   if (PecChk(i*2-1) == SPIData(i*8-1)) && (PecChk(i*2) == SPIData(i*8))
%     DataFault(i) = 1;
%   else
%     DataFault(i) = 0;
%   end
% end



% onemask8 = uint16(hex2dec('00FF'));
% onemask8_8sft = uint16(hex2dec('FF00'));
% onemask88 = uint8(hex2dec('FF'));
% onemask16 = uint16(hex2dec('FFFF'));
%
% % data_test = zeros(1,2);
% remainder = uint16(16);
%
% for i=1:len
%     ii = uint16(i);
% %     data_test(1,i) = data(ii);
% %     address = 2;
%     address = bitand( ...
%         bitxor( ...
%         uint8(bitsra(remainder,7)),data(ii) ), ...
%         onemask88);
%     remainder = bitxor(bitshift(remainder,8,'uint16'),pec15Table(address+1));
% end
% pec15 = uint16(bitand(bitshift(remainder,1,'uint16'),onemask16));
% pec0 = uint8(bitand(pec15,onemask8));
% pec1 = uint8(bitsra(bitand(pec15,onemask8_8sft),8));

== matlab function can_simple_block_bu11143/DataDumpFast1/RawData to StoreData5 ==
  data: StrCell input; CellV_1_104 data_store_memory; VTDataCAN_8b output uint8
function VTDataCAN_8b = fcn(StrCell)
global CellV_1_104;
onemask8 = uint16(hex2dec('00FF'));
onemask8_8sft = uint16(hex2dec('FF00'));
onemask8_56sft = uint64(hex2dec('FF'));
% yl = uint8(bitand(u,onemask8));
% yh = uint8(bitsra(bitand(u,onemask8_8sft),8));
% bitshift(remainder,8)  shift left
% bitsra(remainder,8)  shift right



VTDataCAN_8b =  uint8(zeros(1,8));
VTDataCAN_64b =  uint64(zeros(1,1));
VTDataCAN_4data =  uint8(zeros(1,4));

% VTDataCAN_4data(1) = fix(CellV_1_104(StrCell*4-3)/4);
% VTDataCAN_4data(2) = fix(CellV_1_104(StrCell*4-2)/4);
% VTDataCAN_4data(3) = fix(CellV_1_104(StrCell*4-1)/4);
% VTDataCAN_4data(4) = fix(CellV_1_104(StrCell*4-0)/4);

Bid = StrCell;
VTDataCAN_64b = uint64( Bid ) + ...
                            uint64( bitshift(uint64(CellV_1_104(StrCell*4-3)/4),8 ) ) + ...
                            uint64( bitshift(uint64(CellV_1_104(StrCell*4-2)/4),8+14 ))  + ...
                            uint64( bitshift(uint64(CellV_1_104(StrCell*4-1)/4),8+14+14)  )  + ...
                            uint64( bitshift(uint64(CellV_1_104(StrCell*4-0)/4),8+14+14+14) ) ;

VTDataCAN_8b(1) = uint8( bitand(VTDataCAN_64b,onemask8_56sft) );
VTDataCAN_8b(2) = uint8( bitand(bitsra(VTDataCAN_64b,8*1),onemask8_56sft) );
VTDataCAN_8b(3) = uint8( bitand(bitsra(VTDataCAN_64b,8*2),onemask8_56sft) );
VTDataCAN_8b(4) = uint8( bitand(bitsra(VTDataCAN_64b,8*3),onemask8_56sft) );
VTDataCAN_8b(5) = uint8( bitand(bitsra(VTDataCAN_64b,8*4),onemask8_56sft) );
VTDataCAN_8b(6) = uint8( bitand(bitsra(VTDataCAN_64b,8*5),onemask8_56sft) );
VTDataCAN_8b(7) = uint8( bitand(bitsra(VTDataCAN_64b,8*6),onemask8_56sft) );
VTDataCAN_8b(8) = uint8( bitand(bitsra(VTDataCAN_64b,8*7),onemask8_56sft) );

% VTDataCAN_8b(1) = Bid;
% VTDataCAN_8b(2) = VTDataCAN_4data(1)/(2^8);
% VTDataCAN_8b(3) = 4*fix(mod(CellV_1_104(StrCell*4-3),2^8)/4);
% VTDataCAN_8b(3) = VTDataCAN_8b(3) + CellV_1_104(StrCell*4-2)/(2^14);
% VTDataCAN_8b(4) = mod(CellV_1_104(StrCell*4-2),2^14) / (2^8);
% VTDataCAN_8b(5) =  * fix(mod(CellV_1_104(StrCell*4-2),2^6));

4*fix(CellV_1_104(StrCell*4-3)/4);


% VTDataCAN_8b(1) =         CellV_1_104(StrCell*4-3)/256;
% VTDataCAN_8b(2) = mod(CellV_1_104(StrCell*4-3),256);
% VTDataCAN_8b(3) =         CellV_1_104(StrCell*4-2)/256;
% VTDataCAN_8b(4) = mod(CellV_1_104(StrCell*4-2),256);
% VTDataCAN_8b(5) =         CellV_1_104(StrCell*4-1)/256;
% VTDataCAN_8b(6) = mod(CellV_1_104(StrCell*4-1),256);
% VTDataCAN_8b(7) =         CellV_1_104(StrCell*4   )/256;
% VTDataCAN_8b(8) = mod(CellV_1_104(StrCell*4   ),256);

% VTDataCAN_8b(1) =         CellV_1_104(1)/256;
% VTDataCAN_8b(2) = mod(CellV_1_104(1),256);
% VTDataCAN_8b(3) =         CellV_1_104(2)/256;
% VTDataCAN_8b(4) = mod(CellV_1_104(2),256);
% VTDataCAN_8b(5) =         CellV_1_104(9)/256;
% VTDataCAN_8b(6) = mod(CellV_1_104(9),256);
% VTDataCAN_8b(7) =         CellV_1_104(10)/256;
% VTDataCAN_8b(8) = mod(CellV_1_104(10),256);

% VTDataCAN_8b(1) =         uint16(30000)/256;
% VTDataCAN_8b(2) = mod(uint16(30000),256);
% VTDataCAN_8b(3) =         uint16(35000)/256;
% VTDataCAN_8b(4) = mod(uint16(35000),256);
% VTDataCAN_8b(5) =         uint16(33000)/256;
% VTDataCAN_8b(6) = mod(uint16(33000),256);
% VTDataCAN_8b(7) =         uint16(20000)/256;
% VTDataCAN_8b(8) = mod(uint16(20000),256);


end








% CellV_1_104(1) = uint16(1);

% SPIDataStore = uint16(zeros(1,21));
% DataFault =  zeros(1,7);
%
% for i=1:7
%   SPIDataStore(i*3-2) = SPIData(i*8-7)+SPIData(i*8-6)*256;
%   SPIDataStore(i*3-1) = SPIData(i*8-5)+SPIData(i*8-4)*256;
%   SPIDataStore(i*3   ) = SPIData(i*8-3)+SPIData(i*8-2)*256;
%   if (PecChk(i*2-1) == SPIData(i*8-1)) && (PecChk(i*2) == SPIData(i*8))
%     DataFault(i) = 1;
%   else
%     DataFault(i) = 0;
%   end
% end



% onemask8 = uint16(hex2dec('00FF'));
% onemask8_8sft = uint16(hex2dec('FF00'));
% onemask88 = uint8(hex2dec('FF'));
% onemask16 = uint16(hex2dec('FFFF'));
%
% % data_test = zeros(1,2);
% remainder = uint16(16);
%
% for i=1:len
%     ii = uint16(i);
% %     data_test(1,i) = data(ii);
% %     address = 2;
%     address = bitand( ...
%         bitxor( ...
%         uint8(bitsra(remainder,7)),data(ii) ), ...
%         onemask88);
%     remainder = bitxor(bitshift(remainder,8,'uint16'),pec15Table(address+1));
% end
% pec15 = uint16(bitand(bitshift(remainder,1,'uint16'),onemask16));
% pec0 = uint8(bitand(pec15,onemask8));
% pec1 = uint8(bitsra(bitand(pec15,onemask8_8sft),8));
